simulink model "invent_flow"  (R2019b)
settings: Solver=VariableStepAuto  StartTime=0.0  StopTime=10.0  RelTol=1e-3
settings Model: Creator=Shivu  LastModifiedBy=Shivu

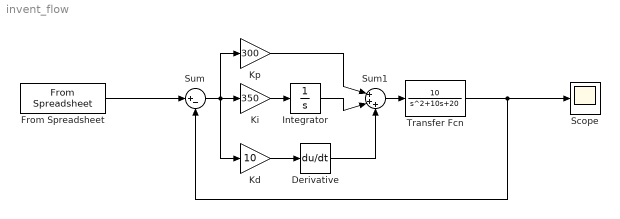
== system invent_flow ==
  Derivative : Derivative
  From Spreadsheet : FromSpreadsheet  FileName=C:\Users\Shivu\Desktop\invent1.xlsx  Range=A2:B88
  Integrator : Integrator
  Kd : Gain  Gain=10
  Ki : Gain  Gain=350
  "Kp " : Gain  Gain=300
  Scope : Scope
  Sum : Sum  Inputs=|+-
  Sum1 : Sum  Inputs=|+++
  Transfer Fcn : TransferFcn  Numerator=[10]  Denominator=[1 10 20]
  wires:
  From Spreadsheet/1 -> Sum/1
  Transfer Fcn/1 -> Sum/2, Scope/1
  Sum/1 -> Kd/1, Ki/1, "Kp "/1
  Sum1/1 -> Transfer Fcn/1
  Ki/1 -> Integrator/1
  Kd/1 -> Derivative/1
  Integrator/1 -> Sum1/2
  Derivative/1 -> Sum1/3
  "Kp "/1 -> Sum1/1
